simulink model "Combined_Experiment_Nov9_2020a"  (R2020a)
settings: Solver=FixedStepAuto  StartTime=0.0  StopTime=tsim  FixedStep=baseRate  RelTol=1e-3  EnableMultiTasking=on
values from neighbouring files (symbols this model uses):
  baseRate = 0.05    [Run_Initializer.m]
  D = 0    [ModelingActuator.m]
  drop_states_ARM = [ pi/2, pi/2, 0]    [Run_Initializer.m]
  drop_states_BLACK = [ xLength/2, yLength/2, pi]    [Run_Initializer.m]
  drop_states_BLUE = [ xLength/2, yLength/2, pi]    [Run_Initializer.m]
  drop_states_RED = [ xLength/2+0.5, yLength/2, pi]    [Run_Initializer.m]
  F_Black_X_nominal = 0.2196    [Run_Initializer.m]
  F_Black_Y_nominal = 0.2825    [Run_Initializer.m]
  F_Blue_X_nominal = 0.2196    [Run_Initializer.m]
  F_Blue_Y_nominal = 0.2825    [Run_Initializer.m]
  F_red_X_nominal = 0.2196    [Run_Initializer.m]
  F_red_Y_nominal = 0.2825    [Run_Initializer.m]
  F_thrusters_BLACK = [F_Black_X_nominal; F_Black_X_nominal;                             F_Black_Y_nominal; F_Black_Y_nominal; F_Black_X_nominal;                              F_Black_X_nominal; F_Black_Y_nominal; F_Black_Y_nominal]    [Run_Initializer.m]
  F_thrusters_BLUE = [F_Blue_X_nominal; F_Blue_X_nominal;                             F_Blue_Y_nominal; F_Blue_Y_nominal; F_Blue_X_nominal;                              F_Blue_X_nominal; F_Blue_Y_nominal; F_Blue_Y_nominal]    [Run_Initializer.m]
  F_thrusters_RED = [F_red_X_nominal; F_red_X_nominal;                             F_red_Y_nominal; F_red_Y_nominal; F_red_X_nominal;                              F_red_X_nominal; F_red_Y_nominal; F_red_Y_nominal]    [Run_Initializer.m]
  Gamma1_el = 0.12    [Run_Initializer.m]
  Gamma1_sh = 0.005    [Run_Initializer.m]
  Gamma1_wr = 0.025    [Run_Initializer.m]
  Gamma2_el = 5    [Run_Initializer.m]
  Gamma2_sh = 15    [Run_Initializer.m]
  Gamma2_wr = 5    [Run_Initializer.m]
  Gamma3_el = 10    [Run_Initializer.m]
  Gamma3_sh = 40    [Run_Initializer.m]
  Gamma3_wr = 40    [Run_Initializer.m]
  Gamma4_el = 0.039    [Run_Initializer.m]
  Gamma4_sh = 0.015    [Run_Initializer.m]
  Gamma4_wr = 0.029    [Run_Initializer.m]
  Gamma5_el = 800    [Run_Initializer.m]
  Gamma5_sh = 800    [Run_Initializer.m]
  Gamma5_wr = 800    [Run_Initializer.m]
  Gamma6_el = 0.000001    (= 1e-06)    [Run_Initializer.m]
  Gamma6_sh = 0.005    [Run_Initializer.m]
  Gamma6_wr = 0.02    [Run_Initializer.m]
  home_states_BLACK = [ xLength/2; yLength/2; 0]    [Run_Initializer.m]
  home_states_BLUE = [ xLength/2; yLength/2; 0]    [Run_Initializer.m]
  home_states_RED = [ xLength/2+0.9; yLength/2; pi]    [Run_Initializer.m]
  init_states_BLACK = [ xLength/2; yLength/2; pi]    [Run_Initializer.m]
  init_states_BLUE = [ xLength/2; yLength/2; pi]    [Run_Initializer.m]
  init_states_RED = [ xLength/2+0.9; yLength/2; pi]    [Run_Initializer.m]
  Kd_tb = 1.0    (= 1)    [Run_Initializer.m]
  Kd_tblue = 1    [Run_Initializer.m]
  Kd_tr = 1.0    (= 1)    [Run_Initializer.m]
  Kd_xb = 8    [Run_Initializer.m]
  Kd_xblue = 8    [Run_Initializer.m]
  Kd_xr = 8    [Run_Initializer.m]
  Kd_yb = 8    [Run_Initializer.m]
  Kd_yblue = 8    [Run_Initializer.m]
  Kd_yr = 8    [Run_Initializer.m]
  Kp = [0.08 0 0 ... (first row only)    [Run_Initializer.m]
  Kp_tb = 0.1    [Run_Initializer.m]
  Kp_tblue = 0.1    [Run_Initializer.m]
  Kp_tr = 0.1    [Run_Initializer.m]
  Kp_xb = 2    [Run_Initializer.m]
  Kp_xblue = 2    [Run_Initializer.m]
  Kp_xr = 2    [Run_Initializer.m]
  Kp_yb = 2    [Run_Initializer.m]
  Kp_yblue = 2    [Run_Initializer.m]
  Kp_yr = 2    [Run_Initializer.m]
  Kv = [0.05 0 0 ... (first row only)    [Run_Initializer.m]
  noise_variance_BLACK = 0    [Run_Initializer.m]
  noise_variance_BLUE = 0    [Run_Initializer.m]
  noise_variance_RED = 0    [Run_Initializer.m]
  Phase0_End = Phase0_Duration    (= 10)    [Run_Initializer.m]
  Phase1_End = Phase0_Duration + Phase1_Duration    (= 15)    [Run_Initializer.m]
  Phase2_End = Phase0_Duration + Phase1_Duration +                                   Phase2_Duration    (= 35)    [Run_Initializer.m]
  Phase3_End = Phase0_Duration + Phase1_Duration +                                   Phase2_Duration + Phase3_Duration    (= 550)    [Run_Initializer.m]
  Phase3_SubPhase1_End = Phase2_End + Phase3_SubPhase1_Duration    (= 155)    [Run_Initializer.m]
  Phase3_SubPhase2_End = Phase2_End + Phase3_SubPhase1_Duration +                                   Phase3_SubPhase2_Duration    (= 165)    [Run_Initializer.m]
  Phase3_SubPhase3_End = Phase2_End + Phase3_SubPhase1_Duration +                                   Phase3_SubPhase2_Duration +                                  Phase3_SubPhase3_Duration    (= 195)    [Run_Initializer.m]
  Phase3_SubPhase4_End = Phase2_End + Phase3_SubPhase1_Duration +                                   Phase3_SubPhase2_Duration +                                  Phase3_SubPhase3_Duration +                                  Phase3_SubPhase4_Duration    [Run_Initializer.m]
  Phase4_End = Phase0_Duration + Phase1_Duration +                                   Phase2_Duration + Phase3_Duration +                                   Phase4_Duration    (= 670)    [Run_Initializer.m]
  Phase5_End = Phase0_Duration + Phase1_Duration +                                   Phase2_Duration + Phase3_Duration +                                   Phase4_Duration + Phase5_Duration    (= 690)    [Run_Initializer.m]
  thruster_dist2CG_BLACK = [83.42;-52.58;55.94;-60.05;54.08;-53.92;77.06;-55.94]    [Run_Initializer.m]
  thruster_dist2CG_BLUE = [73.54;-64.46;81.39;-60.11;64.46;-65.94;54.61;-74.39]    [Run_Initializer.m]
  thruster_dist2CG_RED = [49.92;-78.08;70.46;-63.54;81.08;-50.42;57.44;-75.96]    [Run_Initializer.m]
  Tz_lim_elarm = .1    (= 0.1)    [Run_Initializer.m]
  Tz_lim_sharm = .1    (= 0.1)    [Run_Initializer.m]
  Tz_lim_wrarm = .1    (= 0.1)    [Run_Initializer.m]
  xLength = 3.51155    [Run_Initializer.m]
  yLength = 2.41935    [Run_Initializer.m]
undefined symbols (not defined in the file or in its folder): DiscIntNeverNeededParam, model_param, platformSelection, serverRate, simMode
libraries: dspstat3 x18, raspberrypiBasiclib x10, MainLibrary x8, embdlinuxlib x7, dspsigops x6, simulink x6, mspfiltlib x3, dsparch4 x3, sensehatlib x1
(part 10 of 12)

== system Combined_Experiment_Nov9_2020a/Phase #3: Experiment/Change RED Behavior/Sub-Phase #4/RED+ARM/Transpose Jacobian Controller ==
  Ref : Inport
  q : Inport  Port=2
  qdot : Inport  Port=3
  Arm Controller : Subsystem
  Demux1 : Demux  Outputs=6
  End-Effector Position : MATLAB Function  TreatAsAtomicUnit=on
  Error Signal : Subsystem
  Mux1 : Mux  Inputs=3
  Terminator3 : Terminator
  Terminator4 : Terminator
  Terminator5 : Terminator
  "Transpose Generalized Jacobian " : Subsystem
  Control : Outport  VectorParamsAs1DForOutWhenUnconnected=off
  wires:
  Ref/1 -> Error Signal/1(Reference)
  Demux1/1 -> Terminator3/1
  Demux1/2 -> Terminator4/1
  Demux1/3 -> Terminator5/1
  End-Effector Position/1(y) -> Error Signal/2(Current)
  q/1 -> End-Effector Position/1(q), "Transpose Generalized Jacobian "/1(q)
  qdot/1 -> Arm Controller/3("qdot ")
  Mux1/1 -> Control/1
  "Transpose Generalized Jacobian "/1(J^T) -> Arm Controller/2(Jt)
  Demux1/4 -> Mux1/1
  Error Signal/1(Error) -> Arm Controller/1(ye)
  Arm Controller/1(torque) -> Demux1/1
  Demux1/5 -> Mux1/2
  Demux1/6 -> Mux1/3

== system Combined_Experiment_Nov9_2020a/Phase #4: Return Home/Change BLACK Behavior/Custom Discrete PD (Attitude)/x_dot -> x1/Hold this value ==
  In1 : Inport
  Action Port : ActionPort  ActionPortLabel=if(u1 ~= 0)
  Out1 : Outport  VectorParamsAs1DForOutWhenUnconnected=off
  wires:
  In1/1 -> Out1/1

== system Combined_Experiment_Nov9_2020a/Phase #4: Return Home/Change BLACK Behavior/Custom Discrete PD (X-Position)/x_dot -> x1/Hold this value ==
  In1 : Inport
  Action Port : ActionPort  ActionPortLabel=if(u1 ~= 0)
  Out1 : Outport  VectorParamsAs1DForOutWhenUnconnected=off
  wires:
  In1/1 -> Out1/1

== system Combined_Experiment_Nov9_2020a/Phase #4: Return Home/Change BLACK Behavior/Custom Discrete PD (Y-Position)/x_dot -> x1/Hold this value ==
  In1 : Inport
  Action Port : ActionPort  ActionPortLabel=if(u1 ~= 0)
  Out1 : Outport  VectorParamsAs1DForOutWhenUnconnected=off
  wires:
  In1/1 -> Out1/1

== system Combined_Experiment_Nov9_2020a/Phase #4: Return Home/Change BLUE Behavior/Custom Discrete PD (Attitude)/x_dot -> x1/Hold this value ==
  In1 : Inport
  Action Port : ActionPort  ActionPortLabel=if(u1 ~= 0)
  Out1 : Outport  VectorParamsAs1DForOutWhenUnconnected=off
  wires:
  In1/1 -> Out1/1

== system Combined_Experiment_Nov9_2020a/Phase #4: Return Home/Change BLUE Behavior/Custom Discrete PD (X-Position)/x_dot -> x1/Hold this value ==
  In1 : Inport
  Action Port : ActionPort  ActionPortLabel=if(u1 ~= 0)
  Out1 : Outport  VectorParamsAs1DForOutWhenUnconnected=off
  wires:
  In1/1 -> Out1/1

== system Combined_Experiment_Nov9_2020a/Phase #4: Return Home/Change BLUE Behavior/Custom Discrete PD (Y-Position)/x_dot -> x1/Hold this value ==
  In1 : Inport
  Action Port : ActionPort  ActionPortLabel=if(u1 ~= 0)
  Out1 : Outport  VectorParamsAs1DForOutWhenUnconnected=off
  wires:
  In1/1 -> Out1/1

== system Combined_Experiment_Nov9_2020a/Phase #4: Return Home/Change RED Behavior/Custom Discrete PD (Attitude)/x_dot -> x2/Hold this value ==
  In1 : Inport
  Action Port : ActionPort  ActionPortLabel=if(u1 ~= 0)
  Out1 : Outport  VectorParamsAs1DForOutWhenUnconnected=off
  wires:
  In1/1 -> Out1/1

== system Combined_Experiment_Nov9_2020a/Phase #4: Return Home/Change RED Behavior/Custom Discrete PD (X-Position)/x_dot -> x2/Hold this value ==
  In1 : Inport
  Action Port : ActionPort  ActionPortLabel=if(u1 ~= 0)
  Out1 : Outport  VectorParamsAs1DForOutWhenUnconnected=off
  wires:
  In1/1 -> Out1/1

== system Combined_Experiment_Nov9_2020a/Phase #4: Return Home/Change RED Behavior/Custom Discrete PD (Y-Position)/x_dot -> x2/Hold this value ==
  In1 : Inport
  Action Port : ActionPort  ActionPortLabel=if(u1 ~= 0)
  Out1 : Outport  VectorParamsAs1DForOutWhenUnconnected=off
  wires:
  In1/1 -> Out1/1

== system Combined_Experiment_Nov9_2020a/Phase #4: Return Home/Change RED Behavior/RED+ARM/Transpose Jacobian Controller/Arm Controller ==
  ye : Inport
  Jt : Inport  Port=2
  "qdot " : Inport  Port=3
  MATLAB Function : MATLAB Function  TreatAsAtomicUnit=on
  torque : Outport  VectorParamsAs1DForOutWhenUnconnected=off
  wires:
  ye/1 -> MATLAB Function/1(dx)
  Jt/1 -> MATLAB Function/3(Jt)
  "qdot "/1 -> MATLAB Function/2(qdot)
  MATLAB Function/1(TAU_out) -> torque/1

== system Combined_Experiment_Nov9_2020a/Phase #4: Return Home/Change RED Behavior/RED+ARM/Transpose Jacobian Controller/Error Signal ==
  Reference : Inport
  Current : Inport  Port=2
  End-Effector Position1 : MATLAB Function  Commented=on  TreatAsAtomicUnit=on
  Reshape : Reshape  OutputDimensionality=Row vector (2-D)
  Subtract : Sum  Inputs=+-
  Error : Outport  VectorParamsAs1DForOutWhenUnconnected=off
  wires:
  Subtract/1 -> Error/1
  Current/1 -> Subtract/2
  Reshape/1 -> Subtract/1
  Reference/1 -> Reshape/1

== system Combined_Experiment_Nov9_2020a/Phase #4: Return Home/Change RED Behavior/RED+ARM/Transpose Jacobian Controller/Transpose Generalized Jacobian  ==
  q : Inport
  "Inertia Function " : MATLAB Function  TreatAsAtomicUnit=on
  MATLAB Function : MATLAB Function  TreatAsAtomicUnit=on
  Math Function : Math  Operator=transpose  SignedPower=on  SaturateOnIntegerOverflow=on
  J^T : Outport  VectorParamsAs1DForOutWhenUnconnected=off
  wires:
  Math Function/1 -> J^T/1
  q/1 -> "Inertia Function "/1(x), MATLAB Function/1(q)
  MATLAB Function/1(J) -> Math Function/1
  "Inertia Function "/1(InertiaS) -> MATLAB Function/2(InertiaS)

== system Combined_Experiment_Nov9_2020a/Phase #5: Hold Home/Change BLACK Behavior/Custom Discrete PD (Attitude)/x_dot -> x1/Hold this value ==
  In1 : Inport
  Action Port : ActionPort  ActionPortLabel=if(u1 ~= 0)
  Out1 : Outport  VectorParamsAs1DForOutWhenUnconnected=off
  wires:
  In1/1 -> Out1/1

== system Combined_Experiment_Nov9_2020a/Phase #5: Hold Home/Change BLACK Behavior/Custom Discrete PD (X-Position)/x_dot -> x1/Hold this value ==
  In1 : Inport
  Action Port : ActionPort  ActionPortLabel=if(u1 ~= 0)
  Out1 : Outport  VectorParamsAs1DForOutWhenUnconnected=off
  wires:
  In1/1 -> Out1/1

== system Combined_Experiment_Nov9_2020a/Phase #5: Hold Home/Change BLACK Behavior/Custom Discrete PD (Y-Position)/x_dot -> x1/Hold this value ==
  In1 : Inport
  Action Port : ActionPort  ActionPortLabel=if(u1 ~= 0)
  Out1 : Outport  VectorParamsAs1DForOutWhenUnconnected=off
  wires:
  In1/1 -> Out1/1

== system Combined_Experiment_Nov9_2020a/Phase #5: Hold Home/Change BLUE Behavior/Custom Discrete PD (Attitude)/x_dot -> x1/Hold this value ==
  In1 : Inport
  Action Port : ActionPort  ActionPortLabel=if(u1 ~= 0)
  Out1 : Outport  VectorParamsAs1DForOutWhenUnconnected=off
  wires:
  In1/1 -> Out1/1

== system Combined_Experiment_Nov9_2020a/Phase #5: Hold Home/Change BLUE Behavior/Custom Discrete PD (X-Position)/x_dot -> x1/Hold this value ==
  In1 : Inport
  Action Port : ActionPort  ActionPortLabel=if(u1 ~= 0)
  Out1 : Outport  VectorParamsAs1DForOutWhenUnconnected=off
  wires:
  In1/1 -> Out1/1

== system Combined_Experiment_Nov9_2020a/Phase #5: Hold Home/Change BLUE Behavior/Custom Discrete PD (Y-Position)/x_dot -> x1/Hold this value ==
  In1 : Inport
  Action Port : ActionPort  ActionPortLabel=if(u1 ~= 0)
  Out1 : Outport  VectorParamsAs1DForOutWhenUnconnected=off
  wires:
  In1/1 -> Out1/1

== system Combined_Experiment_Nov9_2020a/Phase #5: Hold Home/Change RED Behavior/Custom Discrete PD (Attitude)/x_dot -> x2/Hold this value ==
  In1 : Inport
  Action Port : ActionPort  ActionPortLabel=if(u1 ~= 0)
  Out1 : Outport  VectorParamsAs1DForOutWhenUnconnected=off
  wires:
  In1/1 -> Out1/1

== system Combined_Experiment_Nov9_2020a/Phase #5: Hold Home/Change RED Behavior/Custom Discrete PD (X-Position)/x_dot -> x2/Hold this value ==
  In1 : Inport
  Action Port : ActionPort  ActionPortLabel=if(u1 ~= 0)
  Out1 : Outport  VectorParamsAs1DForOutWhenUnconnected=off
  wires:
  In1/1 -> Out1/1

== system Combined_Experiment_Nov9_2020a/Phase #5: Hold Home/Change RED Behavior/Custom Discrete PD (Y-Position)/x_dot -> x2/Hold this value ==
  In1 : Inport
  Action Port : ActionPort  ActionPortLabel=if(u1 ~= 0)
  Out1 : Outport  VectorParamsAs1DForOutWhenUnconnected=off
  wires:
  In1/1 -> Out1/1

== system Combined_Experiment_Nov9_2020a/Phase #5: Hold Home/Change RED Behavior/RED+ARM/Transpose Jacobian Controller/Arm Controller ==
  ye : Inport
  Jt : Inport  Port=2
  "qdot " : Inport  Port=3
  MATLAB Function : MATLAB Function  TreatAsAtomicUnit=on
  torque : Outport  VectorParamsAs1DForOutWhenUnconnected=off
  wires:
  ye/1 -> MATLAB Function/1(dx)
  Jt/1 -> MATLAB Function/3(Jt)
  "qdot "/1 -> MATLAB Function/2(qdot)
  MATLAB Function/1(TAU_out) -> torque/1

== system Combined_Experiment_Nov9_2020a/Phase #5: Hold Home/Change RED Behavior/RED+ARM/Transpose Jacobian Controller/Error Signal ==
  Reference : Inport
  Current : Inport  Port=2
  End-Effector Position1 : MATLAB Function  Commented=on  TreatAsAtomicUnit=on
  Reshape : Reshape  OutputDimensionality=Row vector (2-D)
  Subtract : Sum  Inputs=+-
  Error : Outport  VectorParamsAs1DForOutWhenUnconnected=off
  wires:
  Subtract/1 -> Error/1
  Current/1 -> Subtract/2
  Reshape/1 -> Subtract/1
  Reference/1 -> Reshape/1

== system Combined_Experiment_Nov9_2020a/Phase #5: Hold Home/Change RED Behavior/RED+ARM/Transpose Jacobian Controller/Transpose Generalized Jacobian  ==
  q : Inport
  "Inertia Function " : MATLAB Function  TreatAsAtomicUnit=on
  MATLAB Function : MATLAB Function  TreatAsAtomicUnit=on
  Math Function : Math  Operator=transpose  SignedPower=on  SaturateOnIntegerOverflow=on
  J^T : Outport  VectorParamsAs1DForOutWhenUnconnected=off
  wires:
  Math Function/1 -> J^T/1
  q/1 -> "Inertia Function "/1(x), MATLAB Function/1(q)
  MATLAB Function/1(J) -> Math Function/1
  "Inertia Function "/1(InertiaS) -> MATLAB Function/2(InertiaS)

== system Combined_Experiment_Nov9_2020a/Simulate Plant Dynamics/RED and ARM Dynamics/RED + ARM/RED + ARM Dynamics/x_dot -> x1 ==
  note: dy/dt ~= (y2-y1)/deltaT
  y(t) : Inport
  Delay1 : Delay  DelayLength=1  InitialConditionSource=Input port
      settings: InputPortMap=u0,p4
  Hold this value : Subsystem  TreatAsAtomicUnit=on
  Sum6 : Sum  Inputs=-+|
  divide by delta T : Gain  Gain=1/baseRate
  "if we went through a \"step\"" : If  IfExpression=u1 ~= 0  ShowElse=off
  dy(t)/dt : Outport  VectorParamsAs1DForOutWhenUnconnected=off
  wires:
  divide by delta T/1 -> dy(t)/dt/1
  Delay1/1 -> Sum6/1
  "if we went through a \"step\""/1 -> Hold this value/Action
  Hold this value/1(Out1) -> divide by delta T/1
  Sum6/1 -> "if we went through a \"step\""/1, Hold this value/1(In1)
  y(t)/1 -> Sum6/2, Delay1/2, Delay1/1

== system Combined_Experiment_Nov9_2020a/Simulate Plant Dynamics/RED and ARM Dynamics/RED + ARM/RED + ARM Dynamics/x_dot -> x2 ==
  note: dy/dt ~= (y2-y1)/deltaT
  y(t) : Inport
  Delay1 : Delay  DelayLength=1  InitialConditionSource=Input port
      settings: InputPortMap=u0,p4
  Hold this value : Subsystem  TreatAsAtomicUnit=on
  Sum6 : Sum  Inputs=-+|
  divide by delta T : Gain  Gain=1/baseRate
  "if we went through a \"step\"" : If  IfExpression=u1 ~= 0  ShowElse=off
  dy(t)/dt : Outport  VectorParamsAs1DForOutWhenUnconnected=off
  wires:
  divide by delta T/1 -> dy(t)/dt/1
  Delay1/1 -> Sum6/1
  "if we went through a \"step\""/1 -> Hold this value/Action
  Hold this value/1(Out1) -> divide by delta T/1
  Sum6/1 -> "if we went through a \"step\""/1, Hold this value/1(In1)
  y(t)/1 -> Sum6/2, Delay1/2, Delay1/1

== system Combined_Experiment_Nov9_2020a/Simulate Plant Dynamics/RED and ARM Dynamics/RED Only/RED Dynamics/RED Dynamics Model ==
  control_inputs : Inport
  Acceleration to Velocity : DiscreteIntegrator  IntegratorMethod=Integration: Backward Euler  SampleTime=-1  ICPrevOutput=DiscIntNeverNeededParam  ICPrevScaledInput=DiscIntNeverNeededParam
  MATLAB Function : MATLAB Function  TreatAsAtomicUnit=on
  Random Number : RandomNumber  Variance=noise_variance_RED
  Sum : Sum  Inputs=|++
  Velocity to Position : DiscreteIntegrator  IntegratorMethod=Integration: Backward Euler  InitialCondition=drop_states_RED  SampleTime=-1  ICPrevOutput=DiscIntNeverNeededParam  ICPrevScaledInput=DiscIntNeverNeededParam
  states : Outport  VectorParamsAs1DForOutWhenUnconnected=off
  wires:
  control_inputs/1 -> MATLAB Function/1(control_inputs)
  MATLAB Function/1(x_ddot) -> Acceleration to Velocity/1
  Acceleration to Velocity/1 -> Velocity to Position/1
  Velocity to Position/1 -> Sum/1
  Sum/1 -> states/1
  Random Number/1 -> Sum/2

== system Combined_Experiment_Nov9_2020a/Simulate Plant Dynamics/RED and ARM Dynamics/RED Only/RED Dynamics/Sample and Hold Data to Match PhaseSpace (RED) ==
  states : Inport
  Constant : Constant  Value=serverRate
  Data Store Read1 : DataStoreRead  DataStoreName=Univ_Time
  MATLAB Function : MATLAB Function  TreatAsAtomicUnit=on
  Sample and Hold : dspsigops/Sample and Hold  trig=Rising edge  initCond=drop_states_RED  latchinput=off
  "states_hold " : Outport  VectorParamsAs1DForOutWhenUnconnected=off
  wires:
  Data Store Read1/1 -> MATLAB Function/1(TIME)
  Constant/1 -> MATLAB Function/2(SERVER)
  MATLAB Function/1(y) -> Sample and Hold/Trigger
  Sample and Hold/1 -> "states_hold "/1
  states/1 -> Sample and Hold/1

== system Combined_Experiment_Nov9_2020a/Simulate Plant Dynamics/RED and ARM Dynamics/RED Only/RED Dynamics/x_dot -> x1 ==
  note: dy/dt ~= (y2-y1)/deltaT
  y(t) : Inport
  Delay1 : Delay  DelayLength=1  InitialConditionSource=Input port
      settings: InputPortMap=u0,p4
  Hold this value : Subsystem  TreatAsAtomicUnit=on
  Sum6 : Sum  Inputs=-+|
  divide by delta T : Gain  Gain=1/baseRate
  "if we went through a \"step\"" : If  IfExpression=u1 ~= 0  ShowElse=off
  dy(t)/dt : Outport  VectorParamsAs1DForOutWhenUnconnected=off
  wires:
  divide by delta T/1 -> dy(t)/dt/1
  Delay1/1 -> Sum6/1
  "if we went through a \"step\""/1 -> Hold this value/Action
  Hold this value/1(Out1) -> divide by delta T/1
  Sum6/1 -> "if we went through a \"step\""/1, Hold this value/1(In1)
  y(t)/1 -> Sum6/2, Delay1/2, Delay1/1

== system Combined_Experiment_Nov9_2020a/Simulate Plant Dynamics/RED and ARM Dynamics/RED Only/RED Dynamics/x_dot -> x2 ==
  note: dy/dt ~= (y2-y1)/deltaT
  y(t) : Inport
  Delay1 : Delay  DelayLength=1  InitialConditionSource=Input port
      settings: InputPortMap=u0,p4
  Hold this value : Subsystem  TreatAsAtomicUnit=on
  Sum6 : Sum  Inputs=-+|
  divide by delta T : Gain  Gain=1/baseRate
  "if we went through a \"step\"" : If  IfExpression=u1 ~= 0  ShowElse=off
  dy(t)/dt : Outport  VectorParamsAs1DForOutWhenUnconnected=off
  wires:
  divide by delta T/1 -> dy(t)/dt/1
  Delay1/1 -> Sum6/1
  "if we went through a \"step\""/1 -> Hold this value/Action
  Hold this value/1(Out1) -> divide by delta T/1
  Sum6/1 -> "if we went through a \"step\""/1, Hold this value/1(In1)
  y(t)/1 -> Sum6/2, Delay1/2, Delay1/1

== system Combined_Experiment_Nov9_2020a/Simulate Plant Dynamics/RED and ARM Dynamics/RED Only/RED Dynamics/x_dot -> x3 ==
  note: dy/dt ~= (y2-y1)/deltaT
  y(t) : Inport
  Delay1 : Delay  DelayLength=1  InitialConditionSource=Input port
      settings: InputPortMap=u0,p4
  Hold this value : Subsystem  TreatAsAtomicUnit=on
  Sum6 : Sum  Inputs=-+|
  divide by delta T : Gain  Gain=1/baseRate
  "if we went through a \"step\"" : If  IfExpression=u1 ~= 0  ShowElse=off
  dy(t)/dt : Outport  VectorParamsAs1DForOutWhenUnconnected=off
  wires:
  divide by delta T/1 -> dy(t)/dt/1
  Delay1/1 -> Sum6/1
  "if we went through a \"step\""/1 -> Hold this value/Action
  Hold this value/1(Out1) -> divide by delta T/1
  Sum6/1 -> "if we went through a \"step\""/1, Hold this value/1(In1)
  y(t)/1 -> Sum6/2, Delay1/2, Delay1/1

== system Combined_Experiment_Nov9_2020a/Simulate Plant Dynamics/RED and ARM Dynamics/RED Only/RED Dynamics/x_dot -> x4 ==
  note: dy/dt ~= (y2-y1)/deltaT
  y(t) : Inport
  Delay1 : Delay  DelayLength=1  InitialConditionSource=Input port
      settings: InputPortMap=u0,p4
  Hold this value : Subsystem  TreatAsAtomicUnit=on
  Sum6 : Sum  Inputs=-+|
  divide by delta T : Gain  Gain=1/baseRate
  "if we went through a \"step\"" : If  IfExpression=u1 ~= 0  ShowElse=off
  dy(t)/dt : Outport  VectorParamsAs1DForOutWhenUnconnected=off
  wires:
  divide by delta T/1 -> dy(t)/dt/1
  Delay1/1 -> Sum6/1
  "if we went through a \"step\""/1 -> Hold this value/Action
  Hold this value/1(Out1) -> divide by delta T/1
  Sum6/1 -> "if we went through a \"step\""/1, Hold this value/1(In1)
  y(t)/1 -> Sum6/2, Delay1/2, Delay1/1

== system Combined_Experiment_Nov9_2020a/Simulate Plant Dynamics/RED and ARM Dynamics/RED Only/RED Dynamics/x_dot -> x5 ==
  note: dy/dt ~= (y2-y1)/deltaT
  y(t) : Inport
  Delay1 : Delay  DelayLength=1  InitialConditionSource=Input port
      settings: InputPortMap=u0,p4
  Hold this value : Subsystem  TreatAsAtomicUnit=on
  Sum6 : Sum  Inputs=-+|
  divide by delta T : Gain  Gain=1/baseRate
  "if we went through a \"step\"" : If  IfExpression=u1 ~= 0  ShowElse=off
  dy(t)/dt : Outport  VectorParamsAs1DForOutWhenUnconnected=off
  wires:
  divide by delta T/1 -> dy(t)/dt/1
  Delay1/1 -> Sum6/1
  "if we went through a \"step\""/1 -> Hold this value/Action
  Hold this value/1(Out1) -> divide by delta T/1
  Sum6/1 -> "if we went through a \"step\""/1, Hold this value/1(In1)
  y(t)/1 -> Sum6/2, Delay1/2, Delay1/1

== system Combined_Experiment_Nov9_2020a/Phase #3: Experiment/Change BLACK Behavior/Sub-Phase #1/Custom Discrete PD (Attitude)/x_dot -> x1/Hold this value ==
  In1 : Inport
  Action Port : ActionPort  ActionPortLabel=if(u1 ~= 0)
  Out1 : Outport  VectorParamsAs1DForOutWhenUnconnected=off
  wires:
  In1/1 -> Out1/1

== system Combined_Experiment_Nov9_2020a/Phase #3: Experiment/Change BLACK Behavior/Sub-Phase #1/Custom Discrete PD (X-Position)/x_dot -> x1/Hold this value ==
  In1 : Inport
  Action Port : ActionPort  ActionPortLabel=if(u1 ~= 0)
  Out1 : Outport  VectorParamsAs1DForOutWhenUnconnected=off
  wires:
  In1/1 -> Out1/1

== system Combined_Experiment_Nov9_2020a/Phase #3: Experiment/Change BLACK Behavior/Sub-Phase #1/Custom Discrete PD (Y-Position)/x_dot -> x1/Hold this value ==
  In1 : Inport
  Action Port : ActionPort  ActionPortLabel=if(u1 ~= 0)
  Out1 : Outport  VectorParamsAs1DForOutWhenUnconnected=off
  wires:
  In1/1 -> Out1/1

== system Combined_Experiment_Nov9_2020a/Phase #3: Experiment/Change BLACK Behavior/Sub-Phase #2 /Custom Discrete PD (Attitude)/x_dot -> x1/Hold this value ==
  In1 : Inport
  Action Port : ActionPort  ActionPortLabel=if(u1 ~= 0)
  Out1 : Outport  VectorParamsAs1DForOutWhenUnconnected=off
  wires:
  In1/1 -> Out1/1

== system Combined_Experiment_Nov9_2020a/Phase #3: Experiment/Change BLACK Behavior/Sub-Phase #2 /Custom Discrete PD (X-Position)/x_dot -> x1/Hold this value ==
  In1 : Inport
  Action Port : ActionPort  ActionPortLabel=if(u1 ~= 0)
  Out1 : Outport  VectorParamsAs1DForOutWhenUnconnected=off
  wires:
  In1/1 -> Out1/1

== system Combined_Experiment_Nov9_2020a/Phase #3: Experiment/Change BLACK Behavior/Sub-Phase #2 /Custom Discrete PD (Y-Position)/x_dot -> x1/Hold this value ==
  In1 : Inport
  Action Port : ActionPort  ActionPortLabel=if(u1 ~= 0)
  Out1 : Outport  VectorParamsAs1DForOutWhenUnconnected=off
  wires:
  In1/1 -> Out1/1

== system Combined_Experiment_Nov9_2020a/Phase #3: Experiment/Change BLACK Behavior/Sub-Phase #3 /Custom Discrete PD (Attitude)/x_dot -> x1/Hold this value ==
  In1 : Inport
  Action Port : ActionPort  ActionPortLabel=if(u1 ~= 0)
  Out1 : Outport  VectorParamsAs1DForOutWhenUnconnected=off
  wires:
  In1/1 -> Out1/1

== system Combined_Experiment_Nov9_2020a/Phase #3: Experiment/Change BLACK Behavior/Sub-Phase #3 /Custom Discrete PD (X-Position)/x_dot -> x1/Hold this value ==
  In1 : Inport
  Action Port : ActionPort  ActionPortLabel=if(u1 ~= 0)
  Out1 : Outport  VectorParamsAs1DForOutWhenUnconnected=off
  wires:
  In1/1 -> Out1/1

== system Combined_Experiment_Nov9_2020a/Phase #3: Experiment/Change BLACK Behavior/Sub-Phase #3 /Custom Discrete PD (Y-Position)/x_dot -> x1/Hold this value ==
  In1 : Inport
  Action Port : ActionPort  ActionPortLabel=if(u1 ~= 0)
  Out1 : Outport  VectorParamsAs1DForOutWhenUnconnected=off
  wires:
  In1/1 -> Out1/1

== system Combined_Experiment_Nov9_2020a/Phase #3: Experiment/Change BLACK Behavior/Sub-Phase #4/Custom Discrete PD (Attitude)/x_dot -> x1/Hold this value ==
  In1 : Inport
  Action Port : ActionPort  ActionPortLabel=if(u1 ~= 0)
  Out1 : Outport  VectorParamsAs1DForOutWhenUnconnected=off
  wires:
  In1/1 -> Out1/1

== system Combined_Experiment_Nov9_2020a/Phase #3: Experiment/Change BLACK Behavior/Sub-Phase #4/Custom Discrete PD (X-Position)/x_dot -> x1/Hold this value ==
  In1 : Inport
  Action Port : ActionPort  ActionPortLabel=if(u1 ~= 0)
  Out1 : Outport  VectorParamsAs1DForOutWhenUnconnected=off
  wires:
  In1/1 -> Out1/1

== system Combined_Experiment_Nov9_2020a/Phase #3: Experiment/Change BLACK Behavior/Sub-Phase #4/Custom Discrete PD (Y-Position)/x_dot -> x1/Hold this value ==
  In1 : Inport
  Action Port : ActionPort  ActionPortLabel=if(u1 ~= 0)
  Out1 : Outport  VectorParamsAs1DForOutWhenUnconnected=off
  wires:
  In1/1 -> Out1/1

== system Combined_Experiment_Nov9_2020a/Phase #3: Experiment/Change BLUE Behavior/Sub-Phase #1/Custom Discrete PD (Attitude)/x_dot -> x1/Hold this value ==
  In1 : Inport
  Action Port : ActionPort  ActionPortLabel=if(u1 ~= 0)
  Out1 : Outport  VectorParamsAs1DForOutWhenUnconnected=off
  wires:
  In1/1 -> Out1/1

== system Combined_Experiment_Nov9_2020a/Phase #3: Experiment/Change BLUE Behavior/Sub-Phase #1/Custom Discrete PD (X-Position)/x_dot -> x1/Hold this value ==
  In1 : Inport
  Action Port : ActionPort  ActionPortLabel=if(u1 ~= 0)
  Out1 : Outport  VectorParamsAs1DForOutWhenUnconnected=off
  wires:
  In1/1 -> Out1/1

== system Combined_Experiment_Nov9_2020a/Phase #3: Experiment/Change BLUE Behavior/Sub-Phase #1/Custom Discrete PD (Y-Position)/x_dot -> x1/Hold this value ==
  In1 : Inport
  Action Port : ActionPort  ActionPortLabel=if(u1 ~= 0)
  Out1 : Outport  VectorParamsAs1DForOutWhenUnconnected=off
  wires:
  In1/1 -> Out1/1

== system Combined_Experiment_Nov9_2020a/Phase #3: Experiment/Change BLUE Behavior/Sub-Phase #2 /Custom Discrete PD (Attitude)/x_dot -> x1/Hold this value ==
  In1 : Inport
  Action Port : ActionPort  ActionPortLabel=if(u1 ~= 0)
  Out1 : Outport  VectorParamsAs1DForOutWhenUnconnected=off
  wires:
  In1/1 -> Out1/1

== system Combined_Experiment_Nov9_2020a/Phase #3: Experiment/Change BLUE Behavior/Sub-Phase #2 /Custom Discrete PD (X-Position)/x_dot -> x1/Hold this value ==
  In1 : Inport
  Action Port : ActionPort  ActionPortLabel=if(u1 ~= 0)
  Out1 : Outport  VectorParamsAs1DForOutWhenUnconnected=off
  wires:
  In1/1 -> Out1/1

== system Combined_Experiment_Nov9_2020a/Phase #3: Experiment/Change BLUE Behavior/Sub-Phase #2 /Custom Discrete PD (Y-Position)/x_dot -> x1/Hold this value ==
  In1 : Inport
  Action Port : ActionPort  ActionPortLabel=if(u1 ~= 0)
  Out1 : Outport  VectorParamsAs1DForOutWhenUnconnected=off
  wires:
  In1/1 -> Out1/1

== system Combined_Experiment_Nov9_2020a/Phase #3: Experiment/Change BLUE Behavior/Sub-Phase #3 /Custom Discrete PD (Attitude)/x_dot -> x1/Hold this value ==
  In1 : Inport
  Action Port : ActionPort  ActionPortLabel=if(u1 ~= 0)
  Out1 : Outport  VectorParamsAs1DForOutWhenUnconnected=off
  wires:
  In1/1 -> Out1/1

== system Combined_Experiment_Nov9_2020a/Phase #3: Experiment/Change BLUE Behavior/Sub-Phase #3 /Custom Discrete PD (X-Position)/x_dot -> x1/Hold this value ==
  In1 : Inport
  Action Port : ActionPort  ActionPortLabel=if(u1 ~= 0)
  Out1 : Outport  VectorParamsAs1DForOutWhenUnconnected=off
  wires:
  In1/1 -> Out1/1

== system Combined_Experiment_Nov9_2020a/Phase #3: Experiment/Change BLUE Behavior/Sub-Phase #3 /Custom Discrete PD (Y-Position)/x_dot -> x1/Hold this value ==
  In1 : Inport
  Action Port : ActionPort  ActionPortLabel=if(u1 ~= 0)
  Out1 : Outport  VectorParamsAs1DForOutWhenUnconnected=off
  wires:
  In1/1 -> Out1/1

== system Combined_Experiment_Nov9_2020a/Phase #3: Experiment/Change BLUE Behavior/Sub-Phase #4/Custom Discrete PD (Attitude)/x_dot -> x1/Hold this value ==
  In1 : Inport
  Action Port : ActionPort  ActionPortLabel=if(u1 ~= 0)
  Out1 : Outport  VectorParamsAs1DForOutWhenUnconnected=off
  wires:
  In1/1 -> Out1/1

== system Combined_Experiment_Nov9_2020a/Phase #3: Experiment/Change BLUE Behavior/Sub-Phase #4/Custom Discrete PD (X-Position)/x_dot -> x1/Hold this value ==
  In1 : Inport
  Action Port : ActionPort  ActionPortLabel=if(u1 ~= 0)
  Out1 : Outport  VectorParamsAs1DForOutWhenUnconnected=off
  wires:
  In1/1 -> Out1/1

== system Combined_Experiment_Nov9_2020a/Phase #3: Experiment/Change BLUE Behavior/Sub-Phase #4/Custom Discrete PD (Y-Position)/x_dot -> x1/Hold this value ==
  In1 : Inport
  Action Port : ActionPort  ActionPortLabel=if(u1 ~= 0)
  Out1 : Outport  VectorParamsAs1DForOutWhenUnconnected=off
  wires:
  In1/1 -> Out1/1

== system Combined_Experiment_Nov9_2020a/Phase #3: Experiment/Change RED Behavior/Sub-Phase #4/RED+ARM/Transpose Jacobian Controller/Arm Controller ==
  ye : Inport
  Jt : Inport  Port=2
  "qdot " : Inport  Port=3
  MATLAB Function : MATLAB Function  TreatAsAtomicUnit=on
  torque : Outport  VectorParamsAs1DForOutWhenUnconnected=off
  wires:
  ye/1 -> MATLAB Function/1(dx)
  Jt/1 -> MATLAB Function/3(Jt)
  "qdot "/1 -> MATLAB Function/2(qdot)
  MATLAB Function/1(TAU_out) -> torque/1

== system Combined_Experiment_Nov9_2020a/Phase #3: Experiment/Change RED Behavior/Sub-Phase #4/RED+ARM/Transpose Jacobian Controller/Error Signal ==
  Reference : Inport
  Current : Inport  Port=2
  End-Effector Position1 : MATLAB Function  Commented=on  TreatAsAtomicUnit=on
  Reshape : Reshape  OutputDimensionality=Row vector (2-D)
  Subtract : Sum  Inputs=+-
  Error : Outport  VectorParamsAs1DForOutWhenUnconnected=off
  wires:
  Subtract/1 -> Error/1
  Current/1 -> Subtract/2
  Reshape/1 -> Subtract/1
  Reference/1 -> Reshape/1

== system Combined_Experiment_Nov9_2020a/Phase #3: Experiment/Change RED Behavior/Sub-Phase #4/RED+ARM/Transpose Jacobian Controller/Transpose Generalized Jacobian  ==
  q : Inport
  "Inertia Function " : MATLAB Function  TreatAsAtomicUnit=on
  MATLAB Function : MATLAB Function  TreatAsAtomicUnit=on
  Math Function : Math  Operator=transpose  SignedPower=on  SaturateOnIntegerOverflow=on
  J^T : Outport  VectorParamsAs1DForOutWhenUnconnected=off
  wires:
  Math Function/1 -> J^T/1
  q/1 -> "Inertia Function "/1(x), MATLAB Function/1(q)
  MATLAB Function/1(J) -> Math Function/1
  "Inertia Function "/1(InertiaS) -> MATLAB Function/2(InertiaS)

== system Combined_Experiment_Nov9_2020a/Simulate Plant Dynamics/RED and ARM Dynamics/RED + ARM/RED + ARM Dynamics/x_dot -> x1/Hold this value ==
  In1 : Inport
  Action Port : ActionPort  ActionPortLabel=if(u1 ~= 0)
  Out1 : Outport  VectorParamsAs1DForOutWhenUnconnected=off
  wires:
  In1/1 -> Out1/1

== system Combined_Experiment_Nov9_2020a/Simulate Plant Dynamics/RED and ARM Dynamics/RED + ARM/RED + ARM Dynamics/x_dot -> x2/Hold this value ==
  In1 : Inport
  Action Port : ActionPort  ActionPortLabel=if(u1 ~= 0)
  Out1 : Outport  VectorParamsAs1DForOutWhenUnconnected=off
  wires:
  In1/1 -> Out1/1

== system Combined_Experiment_Nov9_2020a/Simulate Plant Dynamics/RED and ARM Dynamics/RED Only/RED Dynamics/x_dot -> x1/Hold this value ==
  In1 : Inport
  Action Port : ActionPort  ActionPortLabel=if(u1 ~= 0)
  Out1 : Outport  VectorParamsAs1DForOutWhenUnconnected=off
  wires:
  In1/1 -> Out1/1

== system Combined_Experiment_Nov9_2020a/Simulate Plant Dynamics/RED and ARM Dynamics/RED Only/RED Dynamics/x_dot -> x2/Hold this value ==
  In1 : Inport
  Action Port : ActionPort  ActionPortLabel=if(u1 ~= 0)
  Out1 : Outport  VectorParamsAs1DForOutWhenUnconnected=off
  wires:
  In1/1 -> Out1/1

== system Combined_Experiment_Nov9_2020a/Simulate Plant Dynamics/RED and ARM Dynamics/RED Only/RED Dynamics/x_dot -> x3/Hold this value ==
  In1 : Inport
  Action Port : ActionPort  ActionPortLabel=if(u1 ~= 0)
  Out1 : Outport  VectorParamsAs1DForOutWhenUnconnected=off
  wires:
  In1/1 -> Out1/1

== system Combined_Experiment_Nov9_2020a/Simulate Plant Dynamics/RED and ARM Dynamics/RED Only/RED Dynamics/x_dot -> x4/Hold this value ==
  In1 : Inport
  Action Port : ActionPort  ActionPortLabel=if(u1 ~= 0)
  Out1 : Outport  VectorParamsAs1DForOutWhenUnconnected=off
  wires:
  In1/1 -> Out1/1

== system Combined_Experiment_Nov9_2020a/Simulate Plant Dynamics/RED and ARM Dynamics/RED Only/RED Dynamics/x_dot -> x5/Hold this value ==
  In1 : Inport
  Action Port : ActionPort  ActionPortLabel=if(u1 ~= 0)
  Out1 : Outport  VectorParamsAs1DForOutWhenUnconnected=off
  wires:
  In1/1 -> Out1/1

== matlab function Combined_Experiment_Nov9_2020a/Phase #3: Experiment/Change BLUE Behavior/Sub-Phase #1/MATLAB Function3 ==
  data: t input; y output; yLength parameter
function y = fcn(t, yLength)

y = -0.85*sin((0.03490659)*t) + yLength/2;

end

== matlab function Combined_Experiment_Nov9_2020a/Phase #3: Experiment/Change BLUE Behavior/Sub-Phase #3 /Hough Control/MATLAB Function2 ==
  data: Oy output; z input; Ox output
function [Oy, Ox]   = C3( z )
%C3 gives the rotation matrix about the z-axis for an angle 'z'
%   z - the angle about the z-axis which you rotate
%   A - the rotation matrix

Ox = [cos(z) sin(z); -sin(z) cos(z)]*[1;0];
Oy = [cos(z) sin(z); -sin(z) cos(z)]*[0;1];
end

== matlab function Combined_Experiment_Nov9_2020a/Phase #3: Experiment/Change BLUE Behavior/Sub-Phase #3 /Hough Control/MATLAB Function3 ==
  data: z input; Ox output
function Ox    = C3( z )
%C3 gives the rotation matrix about the z-axis for an angle 'z'
%   z - the angle about the z-axis which you rotate
%   A - the rotation matrix

Ox = [cos(z) sin(z); -sin(z) cos(z)]*[1;0];
end

== matlab function Combined_Experiment_Nov9_2020a/Phase #3: Experiment/Change BLUE Behavior/Sub-Phase #3 /Hough Control/MATLAB Function4 ==
  data: Oy input; e_out output; e_in input
function e_out = fcn(Oy, e_in)

a = sign(Oy'*e_in);
e_out = -a*norm(e_in);

== matlab function Combined_Experiment_Nov9_2020a/From Force//Torque to PWM Signal/Change BLUE Behavior/Calculate Thruster ON//OFF/Rotate Forces to Inertial/Create Rotation Matrix ==
  data: Rz input; C_Ib output
function C_Ib = RotateFrame(Rz)

C_bI = [  cos(Rz) sin(Rz)
         -sin(Rz) cos(Rz) ];

C_Ib = inv(C_bI);

end

== matlab function Combined_Experiment_Nov9_2020a/Phase #3: Experiment/Change BLUE Behavior/Sub-Phase #3 /MATLAB Function2 ==
  data: t input; x output; xLength parameter
function x = fcn(t, xLength)

x = -0.85*cos((0.03490659)*t) + xLength/2;

end

== matlab function Combined_Experiment_Nov9_2020a/Phase #3: Experiment/Change BLUE Behavior/Sub-Phase #3 /MATLAB Function3 ==
  data: t input; y output; yLength parameter
function y = fcn(t, yLength)

y = -0.85*sin((0.03490659)*t) + yLength/2;

end

== matlab function Combined_Experiment_Nov9_2020a/Phase #3: Experiment/Change BLUE Behavior/Sub-Phase #4/MATLAB Function2 ==
  data: t input; x output; xLength parameter
function x = fcn(t, xLength)

x = -0.85*cos((0.03490659)*t) + xLength/2;

end

== matlab function Combined_Experiment_Nov9_2020a/Phase #3: Experiment/Change BLUE Behavior/Sub-Phase #4/MATLAB Function3 ==
  data: t input; y output; yLength parameter
function y = fcn(t, yLength)

y = -0.85*sin((0.03490659)*t) + yLength/2;

end

== matlab function Combined_Experiment_Nov9_2020a/Phase #5: Hold Home/Change RED Behavior/Hough Control/MATLAB Function2 ==
  data: Oy output; z input; Ox output
function [Oy, Ox]   = C3( z )
%C3 gives the rotation matrix about the z-axis for an angle 'z'
%   z - the angle about the z-axis which you rotate
%   A - the rotation matrix

Ox = [cos(z) sin(z); -sin(z) cos(z)]*[1;0];
Oy = [cos(z) sin(z); -sin(z) cos(z)]*[0;1];
end

== matlab function Combined_Experiment_Nov9_2020a/Phase #5: Hold Home/Change RED Behavior/Hough Control/MATLAB Function3 ==
  data: z input; Ox output
function Ox    = C3( z )
%C3 gives the rotation matrix about the z-axis for an angle 'z'
%   z - the angle about the z-axis which you rotate
%   A - the rotation matrix

Ox = [cos(z) sin(z); -sin(z) cos(z)]*[1;0];
end

== matlab function Combined_Experiment_Nov9_2020a/Phase #5: Hold Home/Change RED Behavior/Hough Control/MATLAB Function4 ==
  data: Oy input; e_out output; e_in input
function e_out = fcn(Oy, e_in)

a = sign(Oy'*e_in);
e_out = -a*norm(e_in);

== matlab function Combined_Experiment_Nov9_2020a/Manipulator Encoder Data/Change Behavior/Correct for dropouts/Correct Dropouts ==
  data: InputRaw input; FixedInput output
function FixedInput  = DropFixer(InputRaw)

    if (InputRaw(1) < -3)
        
        FixedInput = InputRaw(2);
        
    elseif (InputRaw(1) < -3 && InputRaw(2) < -3)
            
        FixedInput = InputRaw(3);    
        
    elseif (InputRaw(1) < -3 && InputRaw(2) < -3 && InputRaw(3) < -3)
            
        FixedInput = InputRaw(4);    
        
    else
        
        FixedInput = InputRaw(1);
        
    end
       
end

== matlab function Combined_Experiment_Nov9_2020a/Manipulator Encoder Data/Change Behavior/Correct for dropouts1/Correct Dropouts ==
  data: InputRaw input; FixedInput output
function FixedInput  = DropFixer(InputRaw)

    if (InputRaw(1) < -3)
        
        FixedInput = InputRaw(2);
        
    elseif (InputRaw(1) < -3 && InputRaw(2) < -3)
            
        FixedInput = InputRaw(3);    
        
    elseif (InputRaw(1) < -3 && InputRaw(2) < -3 && InputRaw(3) < -3)
            
        FixedInput = InputRaw(4);    
        
    else
        
        FixedInput = InputRaw(1);
        
    end
       
end

== matlab function Combined_Experiment_Nov9_2020a/From Force//Torque to PWM Signal/Change BLUE Behavior/Rotate Forces to Body/Create Rotation Matrix ==
  data: Rz input; C_bI output
function C_bI = RotateFrame(Rz)

C_bI = [  cos(Rz) sin(Rz)
         -sin(Rz) cos(Rz) ];

end

== matlab function Combined_Experiment_Nov9_2020a/Manipulator Encoder Data/Change Behavior/Correct for dropouts2/Correct Dropouts ==
  data: InputRaw input; FixedInput output
function FixedInput  = DropFixer(InputRaw)

    if (InputRaw(1) < -3)
        
        FixedInput = InputRaw(2);
        
    elseif (InputRaw(1) < -3 && InputRaw(2) < -3)
            
        FixedInput = InputRaw(3);    
        
    elseif (InputRaw(1) < -3 && InputRaw(2) < -3 && InputRaw(3) < -3)
            
        FixedInput = InputRaw(4);    
        
    else
        
        FixedInput = InputRaw(1);
        
    end
       
end

== matlab function Combined_Experiment_Nov9_2020a/Phase #2: Move to Initial Position/Change BLACK Behavior/Hough Control/MATLAB Function2 ==
  data: Oy output; z input; Ox output
function [Oy, Ox]   = C3( z )
%C3 gives the rotation matrix about the z-axis for an angle 'z'
%   z - the angle about the z-axis which you rotate
%   A - the rotation matrix

Ox = [cos(z) sin(z); -sin(z) cos(z)]*[1;0];
Oy = [cos(z) sin(z); -sin(z) cos(z)]*[0;1];
end

== matlab function Combined_Experiment_Nov9_2020a/Phase #2: Move to Initial Position/Change BLACK Behavior/Hough Control/MATLAB Function3 ==
  data: z input; Ox output
function Ox    = C3( z )
%C3 gives the rotation matrix about the z-axis for an angle 'z'
%   z - the angle about the z-axis which you rotate
%   A - the rotation matrix

Ox = [cos(z) sin(z); -sin(z) cos(z)]*[1;0];
end

== matlab function Combined_Experiment_Nov9_2020a/Phase #2: Move to Initial Position/Change BLACK Behavior/Hough Control/MATLAB Function4 ==
  data: Oy input; e_out output; e_in input
function e_out = fcn(Oy, e_in)

a = sign(Oy'*e_in);
e_out = -a*norm(e_in);

== matlab function Combined_Experiment_Nov9_2020a/From Force//Torque to PWM Signal/Change BLACK Behavior/Calculate Thruster ON//OFF/MATLAB Function ==
  data: H output; thruster_dist2CG_BLACK parameter; F_thrusters_BLACK parameter
function H = MakeH(thruster_dist2CG_BLACK,F_thrusters_BLACK)

Vec1 = [ -1
         -1
          0 
          0
          1
          1
          0
          0 ];
      
Vec2 = [  0
          0
          1
          1
          0
          0
         -1
         -1 ];
     
Vec3 = thruster_dist2CG_BLACK./1000;

Mat1 = [Vec1, Vec2, Vec3]';

Mat2 = diag((F_thrusters_BLACK./2));

H    = Mat1*Mat2;

end

== matlab function Combined_Experiment_Nov9_2020a/Phase #3: Experiment/Change BLACK Behavior/Sub-Phase #4/BLACK_RzD/Wrap1/MATLAB Function ==
  data: u input; wrappedAngle output
function wrappedAngle = wrapAngle(u)

wrappedAngle = atan2(sin(u),cos(u));

end

== matlab function Combined_Experiment_Nov9_2020a/Phase #3: Experiment/Change BLACK Behavior/Sub-Phase #4/BLACK_RzD1/Wrap1/MATLAB Function ==
  data: u input; wrappedAngle output
function wrappedAngle = wrapAngle(u)

wrappedAngle = atan2(sin(u),cos(u));

end

== matlab function Combined_Experiment_Nov9_2020a/From Force//Torque to PWM Signal/Change BLACK Behavior/Calculate Thruster ON//OFF/MATLAB Function1 ==
  data: H output; thruster_dist2CG_BLACK parameter; F_thrusters_BLACK parameter
function H = MakeH(thruster_dist2CG_BLACK,F_thrusters_BLACK)

Vec1 = [ -1
         -1
          0 
          0
          1
          1
          0
          0 ];
      
Vec2 = [  0
          0
          1
          1
          0
          0
         -1
         -1 ];
     
Vec3 = thruster_dist2CG_BLACK./1000;

Mat1 = [Vec1, Vec2, Vec3]';

Mat2 = diag((F_thrusters_BLACK));

H    = Mat1*Mat2;

end

== matlab function Combined_Experiment_Nov9_2020a/From Force//Torque to PWM Signal/Change BLACK Behavior/Calculate Thruster ON//OFF/MATLAB Function2 ==
  data: ThrustPer_Final output; ThrustPer input
function ThrustPer_Final  = ThrusterSat(ThrustPer)

ValveTime       = 0.007;
TControl        = 0.1;
ThrustPer_Final = zeros(8,1);

if max(ThrustPer) > 1
    ThrustPer_Sat = ThrustPer/max(ThrustPer);
else
    ThrustPer_Sat = ThrustPer;
end

for i = 1:8
    if ThrustPer_Sat(i) > ValveTime/TControl 
        ThrustPer_Final(i) = ThrustPer_Sat(i);
    else
        ThrustPer_Final(i) = 0;
    end
end
   

end

== matlab function Combined_Experiment_Nov9_2020a/From Force//Torque to PWM Signal/Change BLACK Behavior/Calculate Thruster ON//OFF/Rotate Forces to Inertial/Create Rotation Matrix ==
  data: Rz input; C_Ib output
function C_Ib = RotateFrame(Rz)

C_bI = [  cos(Rz) sin(Rz)
         -sin(Rz) cos(Rz) ];

C_Ib = inv(C_bI);

end

== matlab function Combined_Experiment_Nov9_2020a/From Force//Torque to PWM Signal/Change BLACK Behavior/Rotate Forces to Body/Create Rotation Matrix ==
  data: Rz input; C_bI output
function C_bI = RotateFrame(Rz)

C_bI = [  cos(Rz) sin(Rz)
         -sin(Rz) cos(Rz) ];

end

== matlab function Combined_Experiment_Nov9_2020a/From Force//Torque to PWM Signal/Change RED Behavior/Calculate Thruster ON//OFF/Control Mixer Archive/MATLAB Function ==
  data: H output; thruster_dist2CG_RED parameter; F_thrusters_RED parameter
function H = MakeH(thruster_dist2CG_RED,F_thrusters_RED)

Vec1 = [ -1
         -1
          0 
          0
          1
          1
          0
          0 ];
      
Vec2 = [  0
          0
          1
          1
          0
          0
         -1
         -1 ];
     
Vec3 = thruster_dist2CG_RED./1000;

Mat1 = [Vec1, Vec2, Vec3]';

Mat2 = diag((F_thrusters_RED./2));

H    = Mat1*Mat2;

end

== matlab function Combined_Experiment_Nov9_2020a/From Force//Torque to PWM Signal/Change RED Behavior/Calculate Thruster ON//OFF/Control Mixer Archive/MATLAB Function1 ==
  data: H output; thruster_dist2CG_RED parameter; F_thrusters_RED parameter
function H = MakeH(thruster_dist2CG_RED,F_thrusters_RED)

Vec1 = [ -1
         -1
          0 
          0
          1
          1
          0
          0 ];
      
Vec2 = [  0
          0
          1
          1
          0
          0
         -1
         -1 ];
     
Vec3 = thruster_dist2CG_RED./1000;

Mat1 = [Vec1, Vec2, Vec3]';

Mat2 = diag((F_thrusters_RED));

H    = Mat1*Mat2;

end

== matlab function Combined_Experiment_Nov9_2020a/From Force//Torque to PWM Signal/Change RED Behavior/Calculate Thruster ON//OFF/Control Mixer Archive/MATLAB Function2 ==
  data: ThrustPer_Final output; ThrustPer input
function ThrustPer_Final  = ThrusterSat(ThrustPer)

ValveTime       = 0.007;
TControl        = 0.1;
ThrustPer_Final = zeros(8,1);

if max(ThrustPer) > 1
    ThrustPer_Sat = ThrustPer/max(ThrustPer);
else
    ThrustPer_Sat = ThrustPer;
end

for i = 1:8
    if ThrustPer_Sat(i) > ValveTime/TControl 
        ThrustPer_Final(i) = ThrustPer_Sat(i);
    else
        ThrustPer_Final(i) = 0;
    end
end
   

end

== matlab function Combined_Experiment_Nov9_2020a/From Force//Torque to PWM Signal/Change RED Behavior/Calculate Thruster ON//OFF/Control Mixer Archive/Rotate Forces to Inertial/Create Rotation Matrix ==
  data: Rz input; C_Ib output
function C_Ib = RotateFrame(Rz)

C_bI = [  cos(Rz) sin(Rz)
         -sin(Rz) cos(Rz) ];

C_Ib = inv(C_bI);

end

== matlab function Combined_Experiment_Nov9_2020a/Simulate Plant Dynamics/RED and ARM Dynamics/RED Only/RED Dynamics/Sample and Hold Data to Match PhaseSpace (RED)/MATLAB Function ==
  data: TIME input; y output; SERVER input
function y = fcn(TIME, SERVER)

if mod(TIME,SERVER) == 0
    y = 1;
else
    y = 0;
end

== matlab function Combined_Experiment_Nov9_2020a/Simulate Plant Dynamics/BLACK Dynamics/Sample and Hold Data to Match PhaseSpace (BLACK)/MATLAB Function ==
  data: TIME input; y output; SERVER input
function y = fcn(TIME, SERVER)

if mod(TIME,SERVER) == 0
    y = 1;
else
    y = 0;
end

== matlab function Combined_Experiment_Nov9_2020a/From Force//Torque to PWM Signal/Change RED Behavior/Rotate Forces to Body/Create Rotation Matrix ==
  data: Rz input; C_bI output
function C_bI = RotateFrame(Rz)

C_bI = [  cos(Rz) sin(Rz)
         -sin(Rz) cos(Rz) ];

end

== matlab function Combined_Experiment_Nov9_2020a/Phase #2: Move to Initial Position/Change RED Behavior/Hough Control/MATLAB Function2 ==
  data: Oy output; z input; Ox output
function [Oy, Ox]   = C3( z )
%C3 gives the rotation matrix about the z-axis for an angle 'z'
%   z - the angle about the z-axis which you rotate
%   A - the rotation matrix

Ox = [cos(z) sin(z); -sin(z) cos(z)]*[1;0];
Oy = [cos(z) sin(z); -sin(z) cos(z)]*[0;1];
end

== matlab function Combined_Experiment_Nov9_2020a/Phase #2: Move to Initial Position/Change RED Behavior/Hough Control/MATLAB Function3 ==
  data: z input; Ox output
function Ox    = C3( z )
%C3 gives the rotation matrix about the z-axis for an angle 'z'
%   z - the angle about the z-axis which you rotate
%   A - the rotation matrix

Ox = [cos(z) sin(z); -sin(z) cos(z)]*[1;0];
end

== matlab function Combined_Experiment_Nov9_2020a/Phase #2: Move to Initial Position/Change RED Behavior/Hough Control/MATLAB Function4 ==
  data: Oy input; e_out output; e_in input
function e_out = fcn(Oy, e_in)

a = sign(Oy'*e_in);
e_out = -a*norm(e_in);

== matlab function Combined_Experiment_Nov9_2020a/Phase #3: Experiment/Change BLACK Behavior/Sub-Phase #4/Hough Control/MATLAB Function2 ==
  data: Oy output; z input; Ox output
function [Oy, Ox]   = C3( z )
%C3 gives the rotation matrix about the z-axis for an angle 'z'
%   z - the angle about the z-axis which you rotate
%   A - the rotation matrix

Ox = [cos(z) sin(z); -sin(z) cos(z)]*[1;0];
Oy = [cos(z) sin(z); -sin(z) cos(z)]*[0;1];
end
